simulink model "DigitalBase"  (Simulink 8.2)
settings: Solver=ode45  StartTime=0.0  StopTime=10  RelTol=1e-3
undefined symbols (not defined in the file or in its folder): get, rcosine
libraries: commsink2 x2, commutil2 x2, commchan3 x1, dspspect3 x1, commrandsrc2 x1, dspswit3 x1, dsparch4 x1, commsynccomp2 x1, dspsigops x1
settings Model: Creator=Yi_Liu  LastModifiedBy=Administrator
settings DataIOCC: SignalLoggingSaveFormat=Dataset
settings OptimizationCC: ExpressionDepthLimit=128
settings DebuggingCC: FcnCallInpInsideContextMsg=EnableAllAsError  StateNameClashWarn=none
settings GRTTargetCC: CombineOutputUpdateFcns=on  GRTInterface=off

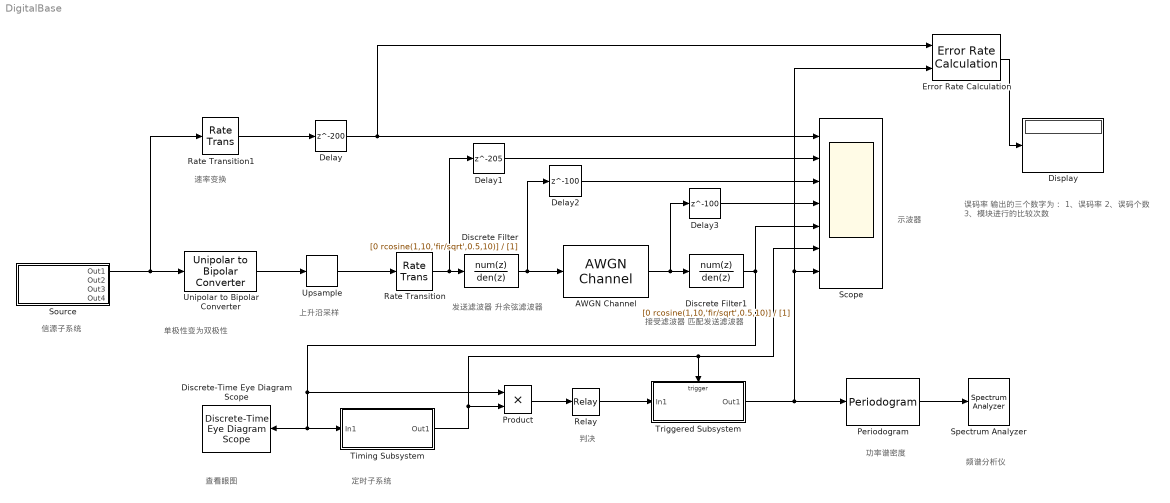
== system DigitalBase ==
  note: 误码率
      | 输出的三个数字为：
      | 1、误码率
      | 2、误码个数
      | 3、模块进行的比较次数
  note: 示波器
  note: 判决
  note: 频谱分析仪
  note: 功率谱密度
  note: 定时子系统
  note: 查看眼图
  note: 接受滤波器
      | 匹配发送滤波器
  note: 发送滤波器
      | 升余弦滤波器
  note: 上升沿采样
  note: 速率变换
  note: 单极性变为双极性
  note: 信源子系统
  AWGN Channel : commchan3/AWGN Channel  InputProcessing=Columns as channels (frame based)  seed=67  noiseMode="Signal to noise ratio  (SNR)"  EbNodB=10  EsNodB=10  SNRdB=10  bitsPerSym=1  Ps=1  Tsym=1  variance=1
  Delay : Delay  DelayLength=200  InitialCondition=0  SampleTime=1/10000
  Delay1 : Delay  DelayLength=205  InitialCondition=0  SampleTime=1/10000
  Delay2 : Delay  DelayLength=100  InitialCondition=0  SampleTime=1/10000
  Delay3 : Delay  DelayLength=100  InitialCondition=0  SampleTime=1/10000
  Discrete Filter : DiscreteFilter  Numerator=[0 rcosine(1,10,'fir/sqrt',0.5,10)]  Denominator=[1]  FilterStructure=Direct form I
  Discrete Filter1 : DiscreteFilter  Numerator=[0 rcosine(1,10,'fir/sqrt',0.5,10)]  Denominator=[1]  FilterStructure=Direct form I
  Discrete-Time Eye Diagram Scope : commsink2/Discrete-Time Eye Diagram Scope  Tag=EyeDiagram  sampPerSymb=50  offsetEye=0  symbPerTrace=1  numTraces=50  numNewFrames=10  LineStyles=-  LineColors=b  dupPoints=on  fading=on  render=on  AxisGrid=on  yMin=-7.82607551428554  yMax=7.98430053144343  inphaseLabel=In-phase Amplitude  quadratureLabel=Quadrature Amplitude  openScopeAtSimStart=on  dispDiagram=In-phase and Quadrature  FrameNumber=off  FigPos=get(0,'defaultfigureposition');  figTitle=Eye Diagram  block_type_=eye  numLinesMax=8
  Display : Display
  Error Rate Calculation : commsink2/Error Rate Calculation  N=0  st_delay=0  cp_mode=Entire frame  subframe=[]  PMode=Port  WsName=ErrorVec  RsMode2=off  stop=off  numErr=100  maxBits=1e6
  Periodogram : dspspect3/Periodogram  measurement=Power spectral density  wintype=Hamming  Rs=50  beta=5  winsamp=Symmetric  FFTImplementation=Auto  inheritFFT=off  fftsize=256  navg=4  inheritTs=on  Ts=1
  Product : Product
  Rate Transition : RateTransition  OutPortSampleTime=1/10000
  Rate Transition1 : RateTransition  OutPortSampleTime=1/10000
  Relay : Relay  OnSwitchValue=0  OffSwitchValue=0  OutDataTypeStr=double
  Scope : Scope  NumInputPorts=7
      settings: YMin=-2~-2~-5~-5~-5~-2~-2  YMax=2~2~5~5~5~2~2
  Source : Subsystem
  Spectrum Analyzer : SpectrumAnalyzer  ScopeSpecification=DataTag1
      settings: CopyFcn=scopeextensions.ScopeBlock.onCoreBlockCopy(gcbh);  DeleteFcn=scopeextensions.ScopeBlock.callback(gcbh, 'onBlockDelete');  PreSaveFcn=scopeextensions.ScopeBlock.callback(gcbh, 'onModelSave');  NameChangeFcn=scopeextensions.ScopeBlock.callback(gcbh, 'onBlockRename');  DestroyFcn=scopeextensions.ScopeBlock.onBlockDestroy(gcbh)  CloseFcn=scopeextensions.ScopeBlock.callback(gcbh, 'onBlockClose');  PreDeleteFcn=scopeextensions.ScopeBlock.callback(gcbh, 'onBlockPreDelete');
  Timing Subsystem : Subsystem
  Triggered Subsystem : Subsystem  TreatAsAtomicUnit=on
  Unipolar to Bipolar Converter : commutil2/Unipolar to Bipolar Converter  M=2  polarity=Positive  dataType=Inherit via internal rule
  Upsample : dspsigops/Upsample  N=2  phase=0  RateOptions=Allow multirate processing  ic=0  mode=Unused parameter value
  wires:
  Upsample/1 -> Rate Transition/1
  Rate Transition/1 -> Discrete Filter/1, Delay1/1
  Discrete Filter/1 -> AWGN Channel/1, Delay2/1
  AWGN Channel/1 -> Delay3/1, Discrete Filter1/1
  Discrete Filter1/1 -> Scope/5, Product/1, Discrete-Time Eye Diagram Scope/1, Timing Subsystem/1(In1)
  Timing Subsystem/1(Out1) -> Scope/6, Triggered Subsystem/Trigger, Product/2
  Product/1 -> Relay/1
  Relay/1 -> Triggered Subsystem/1(In1)
  Rate Transition1/1 -> Delay/1
  Delay/1 -> Error Rate Calculation/1, Scope/1
  Triggered Subsystem/1(Out1) -> Periodogram/1, Error Rate Calculation/2, Scope/7
  Delay2/1 -> Scope/3
  Delay3/1 -> Scope/4
  Delay1/1 -> Scope/2
  Error Rate Calculation/1 -> Display/1
  Periodogram/1 -> Spectrum Analyzer/1
  Source/1(Out1) -> Rate Transition1/1, Unipolar to Bipolar Converter/1
  Unipolar to Bipolar Converter/1 -> Upsample/1

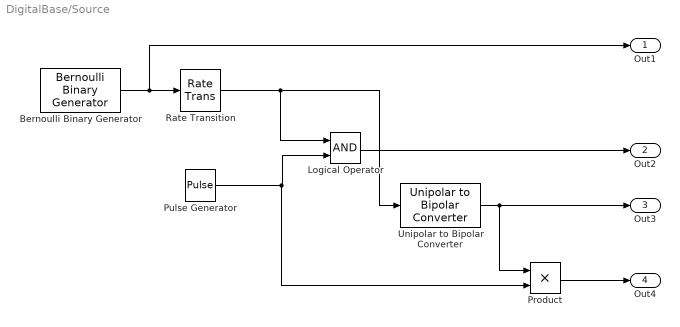
== system DigitalBase/Source ==
  Bernoulli Binary Generator : commrandsrc2/Bernoulli Binary Generator  P=0.5  seed=61  Ts=1/1000  frameBased=off  sampPerFrame=1  orient=off  outDataType=double
  Logical Operator : Logic  AllPortsSameDT=off  OutDataTypeStr=boolean
  Product : Product
  Pulse Generator : DiscretePulseGenerator  Period=10  PulseWidth=5  SampleTime=1/10000
  Rate Transition : RateTransition  OutPortSampleTime=1/10000
  Unipolar to Bipolar Converter : commutil2/Unipolar to Bipolar Converter  M=2  polarity=Positive  dataType=Inherit via internal rule
  Out1 : Outport
  Out2 : Outport  Port=2
  Out3 : Outport  Port=3
  Out4 : Outport  Port=4
  wires:
  Bernoulli Binary Generator/1 -> Out1/1, Rate Transition/1
  Rate Transition/1 -> Logical Operator/1, Unipolar to Bipolar Converter/1
  Pulse Generator/1 -> Product/2, Logical Operator/2
  Unipolar to Bipolar Converter/1 -> Out3/1, Product/1
  Logical Operator/1 -> Out2/1
  Product/1 -> Out4/1

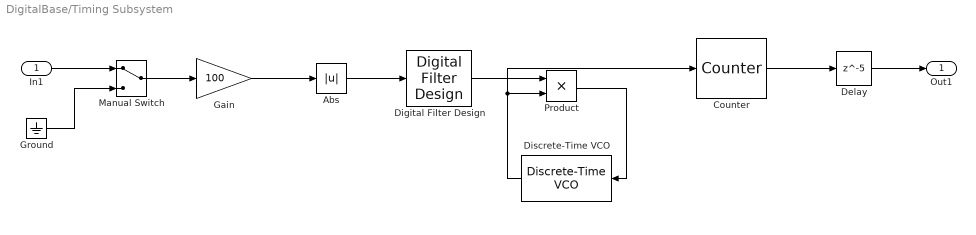
== system DigitalBase/Timing Subsystem ==
  In1 : Inport
  Abs : Abs
  Counter : dspswit3/Counter  Direction=Up  CountEvent=Rising edge  CounterSize=User defined  MaxCount=1  InitialCount=0  Output=Count  HitValue=32  ResetInput=off  SamplesPerFrame=1  Ts=1  CntDtype=int16  HitDtype=Logical
  Delay : Delay  DelayLength=5  SampleTime=1/10000
  Digital Filter Design : dsparch4/Digital Filter Design  mwdsp_browser_bugfix_var=off
  Discrete-Time VCO : commsynccomp2/Discrete-Time VCO  Ac=1  Fc=1994  Kc=8  Ph=0  ts=1/10000
  Gain : Gain  Gain=100
  Ground : Ground
  Manual Switch : ManualSwitch
  Product : Product
  Out1 : Outport
  wires:
  In1/1 -> Manual Switch/1
  Ground/1 -> Manual Switch/2
  Manual Switch/1 -> Gain/1
  Gain/1 -> Abs/1
  Digital Filter Design/1 -> Product/1
  Product/1 -> Discrete-Time VCO/1
  Discrete-Time VCO/1 -> Counter/1, Product/2
  Counter/1 -> Delay/1
  Delay/1 -> Out1/1
  Abs/1 -> Digital Filter Design/1

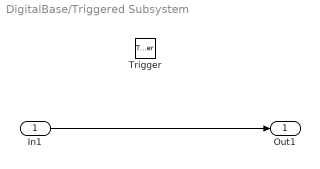
== system DigitalBase/Triggered Subsystem ==
  In1 : Inport
  Trigger : TriggerPort
  Out1 : Outport
  wires:
  In1/1 -> Out1/1
